simulink model "ANTIGOcontrolador"  (R2021a)
settings: Solver=ode23t  StartTime=0.0  StopTime=60  MaxStep=1e-3  RelTol=1e-3
values from neighbouring files (symbols this model uses):
  AL = double(subs(A_par))    [ANTImodeloMATEMATICOFINAL.m]
  BL = double(subs(B_par))    [ANTImodeloMATEMATICOFINAL.m]
  Blo = 8.18575752786119e-06    (= 8.18575752786e-06)    [ANTImodeloMATEMATICOFINAL.m]
  Bmo = 2.02156082362446e-07    (= 2.02156082362e-07)    [ANTImodeloMATEMATICOFINAL.m]
  CL = double(subs(C_par))    [ANTImodeloMATEMATICOFINAL.m]
  DL = double(subs(D_par))    [ANTImodeloMATEMATICOFINAL.m]
  do = 0.06862-0.021    (= 0.04762)    [ANTImodeloMATEMATICOFINAL.m]
  go = 9.81    [ANTImodeloMATEMATICOFINAL.m]
  Jlo = 0.00100697016255642    (= 0.00100697016256)    [ANTImodeloMATEMATICOFINAL.m]
  Jmo = 2.08549279330578e-07    (= 2.08549279331e-07)    [ANTImodeloMATEMATICOFINAL.m]
  Kes = K(:,1:n)    [ANTImodeloMATEMATICOFINAL.m]
  Ki = -K(:,n+1:end)    [ANTImodeloMATEMATICOFINAL.m]
  Kio = 0.00119530882984502    (= 0.00119530882985)    [ANTImodeloMATEMATICOFINAL.m]
  Kvo = 0.0035694528924319    (= 0.00356945289243)    [ANTImodeloMATEMATICOFINAL.m]
  Lo = 0.667669785204658    (= 0.667669785205)    [ANTImodeloMATEMATICOFINAL.m]
  mo = 0.17244    [ANTImodeloMATEMATICOFINAL.m]
  no = 120    [ANTImodeloMATEMATICOFINAL.m]
  Ro = 5.15610211779038    (= 5.15610211779)    [ANTImodeloMATEMATICOFINAL.m]
  Tm = 0.03    [ANTImodeloMATEMATICOFINAL.m]
  Vin0 = Ro*X10    (= 0)    [ANTImodeloMATEMATICOFINAL.m]
  X10 = 0    [ANTImodeloMATEMATICOFINAL.m]
  X20 = 0    [ANTImodeloMATEMATICOFINAL.m]
  X30 = 0    [ANTImodeloMATEMATICOFINAL.m]
libraries: cstblocks x6, slpidlib x4
(part 1 of 2)
settings Model: Creator=hubertdelgado  LastModifiedBy=hubertdelgado

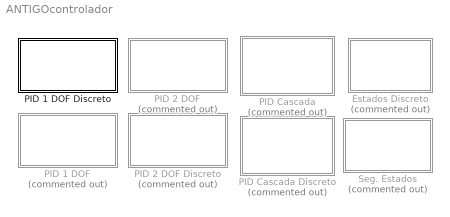
== system ANTIGOcontrolador ==
  Estados Discreto : Subsystem  Commented=on
  "PID 1 DOF " : Subsystem  Commented=on
  PID 1 DOF Discreto : Subsystem
  PID 2 DOF : Subsystem  Commented=on
  PID 2 DOF Discreto : Subsystem  Commented=on
  PID Cascada : Subsystem  Commented=on
  PID Cascada Discreto : Subsystem  Commented=on
  Seg. Estados : Subsystem  Commented=on

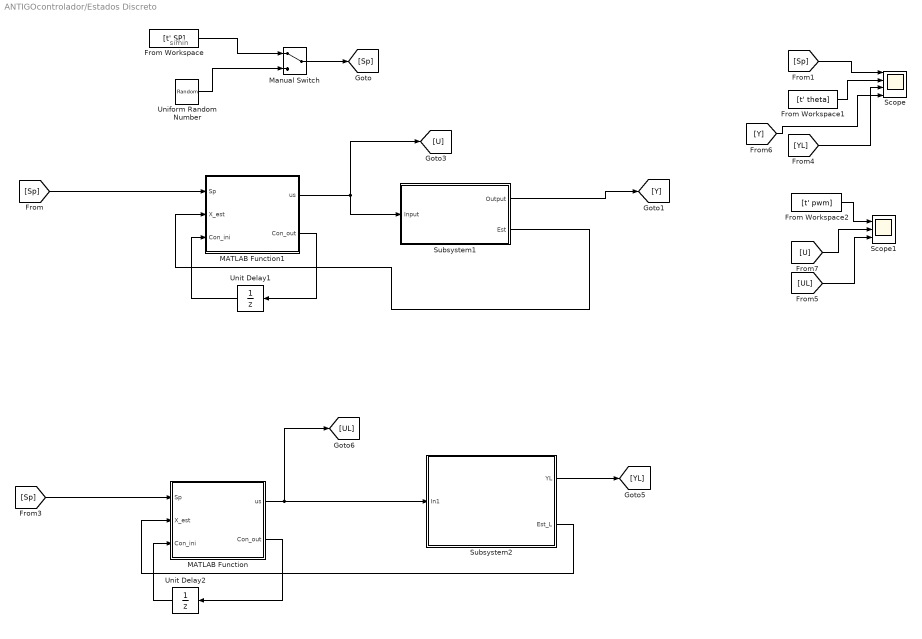
== system ANTIGOcontrolador/Estados Discreto ==
  note: simin
  From Workspace : FromWorkspace  VariableName=[t' SP]
  From Workspace1 : FromWorkspace  VariableName=[t' theta]
  From Workspace2 : FromWorkspace  VariableName=[t' pwm]
  MATLAB Function : MATLAB Function  TreatAsAtomicUnit=on
  MATLAB Function1 : MATLAB Function  TreatAsAtomicUnit=on
  Manual Switch : ManualSwitch
  Scope : Scope  NumInputPorts=4
  Scope1 : Scope  NumInputPorts=3
  Subsystem1 : Subsystem
  Subsystem2 : Subsystem
  Uniform Random Number : UniformRandomNumber  Minimum=-120*(pi/180)  Maximum=120*(pi/180)  SampleTime=10
  Unit Delay1 : UnitDelay  InitialCondition=zeros(1,2)  SampleTime=Tm  HasFrameUpgradeWarning=on
  Unit Delay2 : UnitDelay  InitialCondition=zeros(1,2)  SampleTime=Tm  HasFrameUpgradeWarning=on
  wires:
  Subsystem1/1(Output) -> [Y]
  MATLAB Function/1(us) -> Subsystem2/1(In1), [UL]
  [Sp] -> MATLAB Function/1(Sp)
  MATLAB Function/2(Con_out) -> Unit Delay2/1
  Unit Delay2/1 -> MATLAB Function/3(Con_ini)
  Subsystem2/2(Est_L) -> MATLAB Function/2(X_est)
  Subsystem2/1(YL) -> [YL]
  Manual Switch/1 -> [Sp]
  [Y] -> Scope/4
  From Workspace2/1 -> Scope1/1
  From Workspace/1 -> Manual Switch/1
  From Workspace1/1 -> Scope/2
  Uniform Random Number/1 -> Manual Switch/2
  [Sp] -> Scope/1
  [UL] -> Scope1/3
  [U] -> Scope1/2
  [YL] -> Scope/3
  Subsystem1/2(Est) -> MATLAB Function1/2(X_est)
  Unit Delay1/1 -> MATLAB Function1/3(Con_ini)
  MATLAB Function1/2(Con_out) -> Unit Delay1/1
  [Sp] -> MATLAB Function1/1(Sp)
  MATLAB Function1/1(us) -> [U], Subsystem1/1(Input)

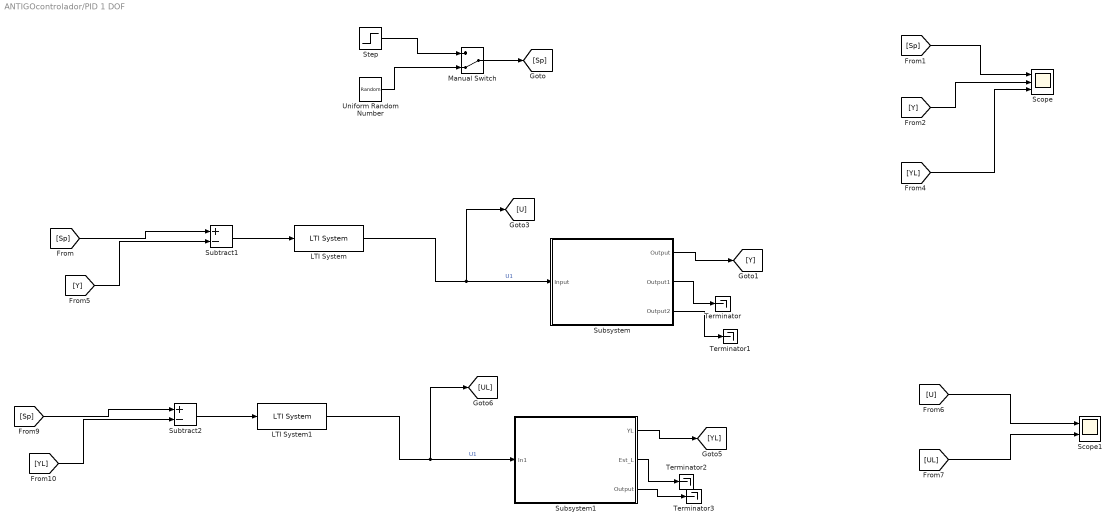
== system ANTIGOcontrolador/PID 1 DOF  ==
  LTI System : cstblocks/LTI System  sys=Cpids  IC=[]
  LTI System1 : cstblocks/LTI System  sys=Cpids  IC=[]
  Manual Switch : ManualSwitch  CurrentSetting=0
  Scope : Scope  NumInputPorts=3
  Scope1 : Scope  NumInputPorts=2
  Step : Step  Time=0  After=0  SampleTime=0
  Subsystem : Subsystem
  Subsystem1 : Subsystem
  Subtract1 : Sum  Inputs=+-
  Subtract2 : Sum  Inputs=+-
  Terminator{,1..3} (4 alike) : Terminator
  Uniform Random Number : UniformRandomNumber  Minimum=-70*(pi/180)  Maximum=70*(pi/180)  SampleTime=10
  wires:
  Manual Switch/1 -> [Sp]
  Uniform Random Number/1 -> Manual Switch/2
  [U] -> Scope1/1
  [UL] -> Scope1/2
  Step/1 -> Manual Switch/1
  Subtract1/1 -> LTI System/1
  LTI System/1 -> Subsystem/1(Input), [U]  "U1"
  [Sp] -> Subtract1/1
  [Y] -> Subtract1/2
  Subsystem/1(Output) -> [Y]
  Subtract2/1 -> LTI System1/1
  [YL] -> Subtract2/2
  LTI System1/1 -> Subsystem1/1(In1), [UL]  "U1"
  Subsystem1/2(Est_L) -> Terminator2/1
  Subsystem1/1(YL) -> [YL]
  [Sp] -> Subtract2/1
  [Sp] -> Scope/1
  [Y] -> Scope/2
  [YL] -> Scope/3
  Subsystem/2(Output1) -> Terminator/1
  Subsystem/3(Output2) -> Terminator1/1
  Subsystem1/3(Output) -> Terminator3/1

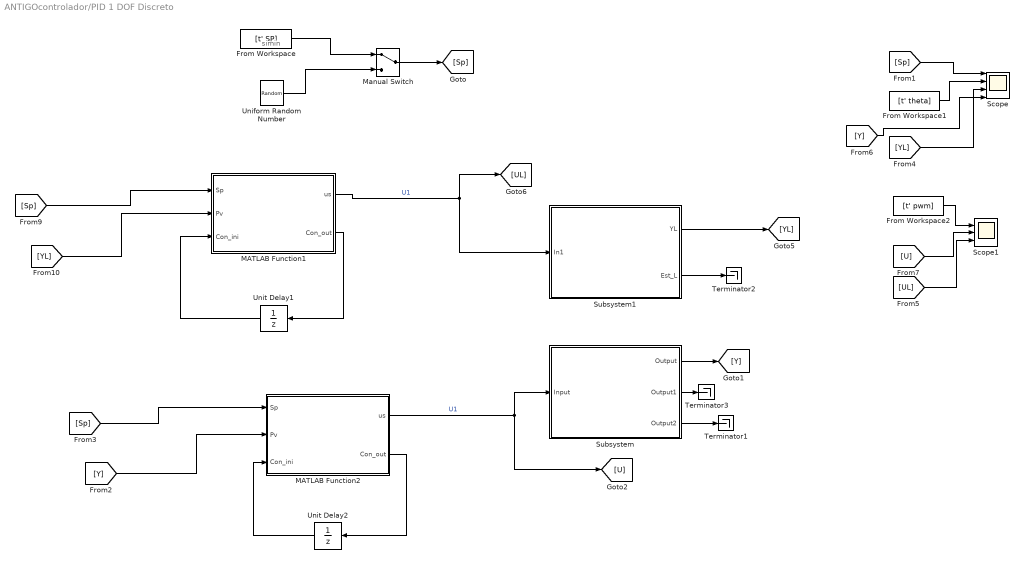
== system ANTIGOcontrolador/PID 1 DOF Discreto ==
  note: simin
  From Workspace : FromWorkspace  VariableName=[t' SP]
  From Workspace1 : FromWorkspace  VariableName=[t' theta]
  From Workspace2 : FromWorkspace  VariableName=[t' pwm]
  MATLAB Function1 : MATLAB Function  TreatAsAtomicUnit=on
  MATLAB Function2 : MATLAB Function  TreatAsAtomicUnit=on
  Manual Switch : ManualSwitch
  Scope : Scope  NumInputPorts=4
  Scope1 : Scope  NumInputPorts=3
  Subsystem : Subsystem
  Subsystem1 : Subsystem
  Terminator1 : Terminator
  Terminator2 : Terminator
  Terminator3 : Terminator
  Uniform Random Number : UniformRandomNumber  Minimum=-60*(pi/180)  Maximum=60*(pi/180)  SampleTime=10
  Unit Delay1 : UnitDelay  InitialCondition=zeros(4,1)  SampleTime=Tm  HasFrameUpgradeWarning=on
  Unit Delay2 : UnitDelay  InitialCondition=zeros(5,1)  SampleTime=Tm  HasFrameUpgradeWarning=on
  wires:
  Manual Switch/1 -> [Sp]
  Uniform Random Number/1 -> Manual Switch/2
  From Workspace2/1 -> Scope1/1
  [U] -> Scope1/2
  From Workspace/1 -> Manual Switch/1
  [YL] -> MATLAB Function1/2(Pv)
  MATLAB Function1/1(us) -> Subsystem1/1(In1), [UL]  "U1"
  Subsystem1/2(Est_L) -> Terminator2/1
  Subsystem1/1(YL) -> [YL]
  [Sp] -> Scope/1
  From Workspace1/1 -> Scope/2
  [YL] -> Scope/3
  Unit Delay1/1 -> MATLAB Function1/3(Con_ini)
  [Sp] -> MATLAB Function1/1(Sp)
  MATLAB Function1/2(Con_out) -> Unit Delay1/1
  Unit Delay2/1 -> MATLAB Function2/3(Con_ini)
  MATLAB Function2/2(Con_out) -> Unit Delay2/1
  MATLAB Function2/1(us) -> [U], Subsystem/1(Input)  "U1"
  [Sp] -> MATLAB Function2/1(Sp)
  [Y] -> MATLAB Function2/2(Pv)
  Subsystem/1(Output) -> [Y]
  Subsystem/3(Output2) -> Terminator1/1
  Subsystem/2(Output1) -> Terminator3/1
  [UL] -> Scope1/3
  [Y] -> Scope/4

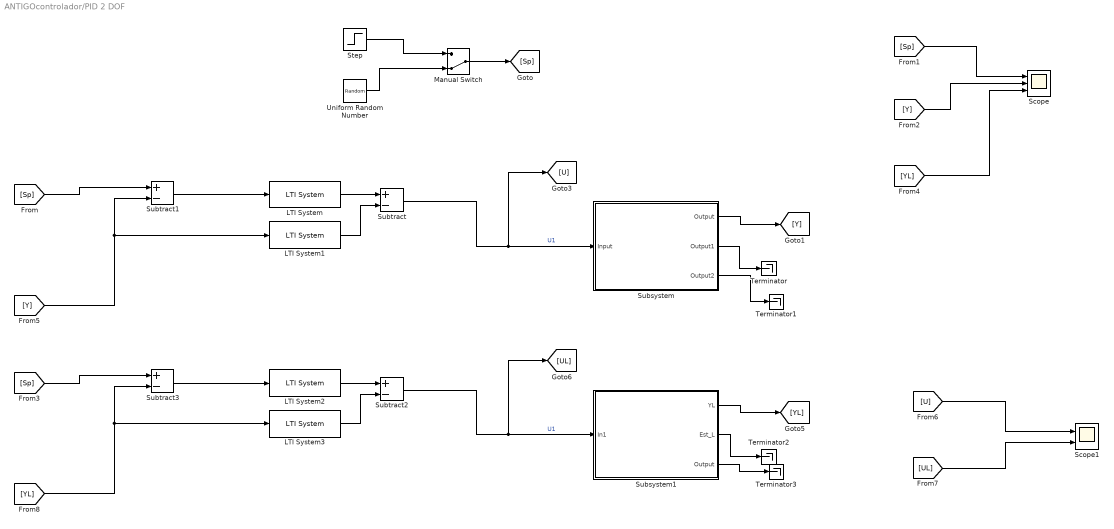
== system ANTIGOcontrolador/PID 2 DOF ==
  LTI System : cstblocks/LTI System  sys=C1s  IC=[]
  LTI System1 : cstblocks/LTI System  sys=C2s  IC=[]
  LTI System2 : cstblocks/LTI System  sys=C1s  IC=[]
  LTI System3 : cstblocks/LTI System  sys=C2s  IC=[]
  Manual Switch : ManualSwitch  CurrentSetting=0
  Scope : Scope  NumInputPorts=3
  Scope1 : Scope  NumInputPorts=2
  Step : Step  Time=0  After=0  SampleTime=0
  Subsystem : Subsystem
  Subsystem1 : Subsystem
  Subtract{,1..3} (4 alike) : Sum  Inputs=+-
  Terminator{,1..3} (4 alike) : Terminator
  Uniform Random Number : UniformRandomNumber  Minimum=-60*(pi/180)  Maximum=60*(pi/180)  SampleTime=10
  wires:
  LTI System/1 -> Subtract/1
  Subtract1/1 -> LTI System/1
  [Sp] -> Subtract1/1
  [Y] -> LTI System1/1, Subtract1/2
  LTI System1/1 -> Subtract/2
  Subtract2/1 -> Subsystem1/1(In1), [UL]  "U1"
  Subsystem1/3(Output) -> Terminator3/1
  Subtract/1 -> Subsystem/1(Input), [U]  "U1"
  Subsystem1/2(Est_L) -> Terminator2/1
  Subsystem/3(Output2) -> Terminator1/1
  Subsystem1/1(YL) -> [YL]
  Subsystem/2(Output1) -> Terminator/1
  Subsystem/1(Output) -> [Y]
  [Sp] -> Subtract3/1
  LTI System3/1 -> Subtract2/2
  LTI System2/1 -> Subtract2/1
  Subtract3/1 -> LTI System2/1
  [YL] -> LTI System3/1, Subtract3/2
  [UL] -> Scope1/2
  Step/1 -> Manual Switch/1
  Manual Switch/1 -> [Sp]
  [Y] -> Scope/2
  [Sp] -> Scope/1
  [YL] -> Scope/3
  [U] -> Scope1/1
  Uniform Random Number/1 -> Manual Switch/2

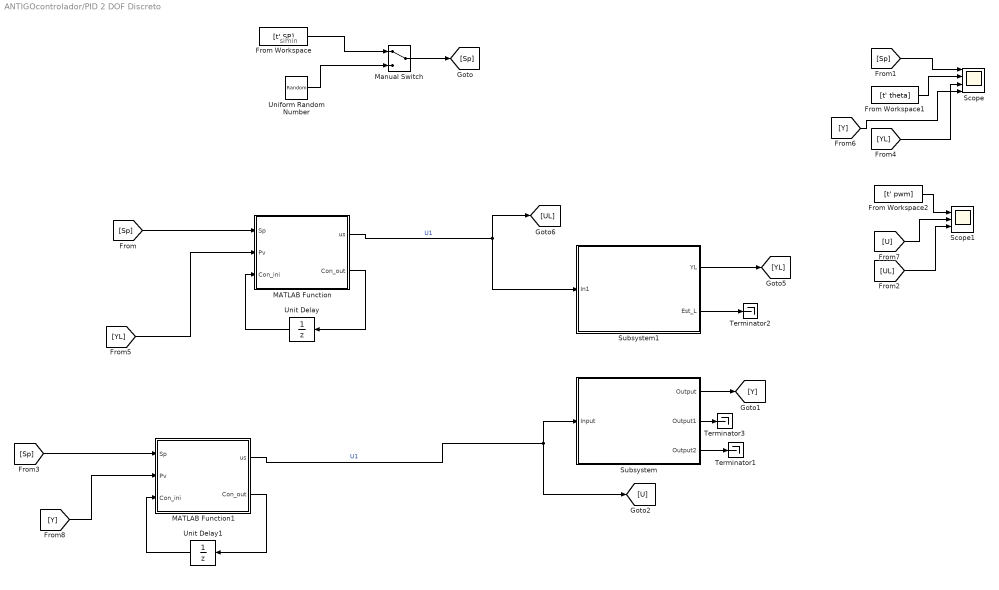
== system ANTIGOcontrolador/PID 2 DOF Discreto ==
  note: simin
  From Workspace : FromWorkspace  VariableName=[t' SP]
  From Workspace1 : FromWorkspace  VariableName=[t' theta]
  From Workspace2 : FromWorkspace  VariableName=[t' pwm]
  MATLAB Function : MATLAB Function  TreatAsAtomicUnit=on
  MATLAB Function1 : MATLAB Function  TreatAsAtomicUnit=on
  Manual Switch : ManualSwitch
  Scope : Scope  NumInputPorts=4
  Scope1 : Scope  NumInputPorts=3
  Subsystem : Subsystem
  Subsystem1 : Subsystem
  Terminator1 : Terminator
  Terminator2 : Terminator
  Terminator3 : Terminator
  Uniform Random Number : UniformRandomNumber  Minimum=-65*(pi/180)  Maximum=65*(pi/180)  SampleTime=10
  Unit Delay : UnitDelay  InitialCondition=zeros(6,1)  SampleTime=Tm  HasFrameUpgradeWarning=on
  Unit Delay1 : UnitDelay  InitialCondition=zeros(6,1)  SampleTime=Tm  HasFrameUpgradeWarning=on
  wires:
  [Sp] -> MATLAB Function/1(Sp)
  Unit Delay/1 -> MATLAB Function/3(Con_ini)
  MATLAB Function/2(Con_out) -> Unit Delay/1
  From Workspace1/1 -> Scope/2
  [YL] -> Scope/3
  [UL] -> Scope1/3
  [U] -> Scope1/2
  [Sp] -> Scope/1
  Uniform Random Number/1 -> Manual Switch/2
  From Workspace/1 -> Manual Switch/1
  From Workspace2/1 -> Scope1/1
  Manual Switch/1 -> [Sp]
  [Y] -> Scope/4
  Subsystem/2(Output1) -> Terminator3/1
  MATLAB Function/1(us) -> Subsystem1/1(In1), [UL]  "U1"
  Subsystem1/2(Est_L) -> Terminator2/1
  Subsystem1/1(YL) -> [YL]
  Subsystem/3(Output2) -> Terminator1/1
  Subsystem/1(Output) -> [Y]
  MATLAB Function1/1(us) -> [U], Subsystem/1(Input)  "U1"
  [Sp] -> MATLAB Function1/1(Sp)
  Unit Delay1/1 -> MATLAB Function1/3(Con_ini)
  MATLAB Function1/2(Con_out) -> Unit Delay1/1
  [YL] -> MATLAB Function/2(Pv)
  [Y] -> MATLAB Function1/2(Pv)

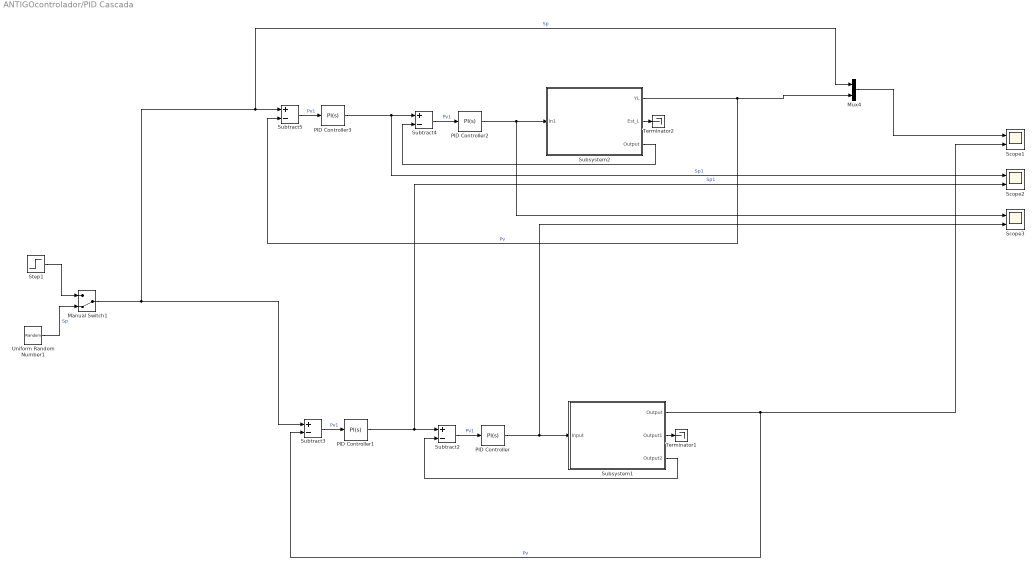
== system ANTIGOcontrolador/PID Cascada ==
  Manual Switch1 : ManualSwitch  CurrentSetting=0
  Mux4 : Mux  Inputs=2
  PID Controller : slpidlib/PID Controller  Controller=PI  Form=Parallel  TimeDomain=Continuous-time  UseExternalTs=off  SampleTime=-1  IntegratorMethod=Forward Euler  FilterMethod=Forward Euler  ControllerParametersSource=internal  P=0.439531738224972  I=0.0931065859182185  D=35.8399189335653  UseFilter=on  N=15672.9006565225  TunerSelectOption=Transfer Function Based (PID Tuner App)  InitialConditionSource=internal  InitialConditionForIntegrator=0  InitialConditionForFilter=0  DifferentiatorICPrevScaledInput=0  ExternalReset=none  TrackingMode=off  Kt=1  LimitOutput=on  SatLimitsSource=internal  UpperSaturationLimit=100  LowerSaturationLimit=-100  LinearizeAsGain=on  AntiWindupMode=none  Kb=1  POutMin=[]  POutMax=[]  IOutMin=[]  IOutMax=[]  DOutMin=[]  DOutMax=[]  NOutMin=[]  NOutMax=[]  SumOutMin=[]  SumOutMax=[]  SaturationOutMin=[]  SaturationOutMax=[]  PParamMin=[]  PParamMax=[]  IParamMin=[]  IParamMax=[]  DParamMin=[]  DParamMax=[]  NParamMin=[]  NParamMax=[]  KbParamMin=[]  KbParamMax=[]  KtParamMin=[]  KtParamMax=[]  KbOutMin=[]  KbOutMax=[]  KtOutMin=[]  KtOutMax=[]  IntegratorOutMin=[]  IntegratorOutMax=[]  FilterOutMin=[]  FilterOutMax=[]  SumI1OutMin=[]  SumI1OutMax=[]  SumI2OutMin=[]  SumI2OutMax=[]  SumI3OutMin=[]  SumI3OutMax=[]  SumI4OutMin=[]  SumI4OutMax=[]  SumDOutMin=[]  SumDOutMax=[]  DifferentiatorOutMin=[]  DifferentiatorOutMax=[]  FilterDiffOutCoefMin=[]  FilterDiffOutCoefMax=[]  ReciprocalOutMin=[]  ReciprocalOutMax=[]  SumDenOutMin=[]  SumDenOutMax=[]  SumNumOutMin=[]  SumNumOutMax=[]  DivideOutMin=[]  DivideOutMax=[]  UdiffTsProdOutMin=[]  UdiffTsProdOutMax=[]  NTsProdOutMin=[]  NTsProdOutMax=[]  UintegralTsProdOutMin=[]  UintegralTsProdOutMax=[]  UngainTsProdOutMin=[]  UngainTsProdOutMax=[]  IntegratorContinuousStateAttributes=''  IntegratorStateMustResolveToSignalObject=off  IntegratorRTWStateStorageClass=Auto  FilterContinuousStateAttributes=''  FilterStateMustResolveToSignalObject=off  FilterRTWStateStorageClass=Auto  ParallelPVariant=InternalParameters  IdealPVariant=Disabled  IVariant=InternalParameters  DVariant=Disabled  IntegratorVariant=Continuous  SatVariant=Enabled  AWVariant=Passthrough  PCopyVariant=Disabled  TRVariant=Disabled  FdbkBlocksVariant=Forward  IdealPFdbkVariant=Disabled  SatFdbkVariant=Disabled  DerivativeFilterVariant=Disabled  NVariant=Disabled  NCopyVariant=Disabled_SignalSpec  FilterICVariant=Disabled  IntegratorICVariant=InternalICs  ExternalResetVariant=Disabled  TRSumVariant=Passthrough  SumFdbkVariant=Disabled  SumVariant=Sum_PI  TsampFilterVariant=InternalTs  TsampNgainVariant=Passthrough  TsampIntegralVariant=Passthrough  ExternalSaturationOutDataTypeStr=Inherit: Same as second input
  PID Controller1 : slpidlib/PID Controller  Controller=PI  Form=Parallel  TimeDomain=Continuous-time  UseExternalTs=off  SampleTime=-1  IntegratorMethod=Forward Euler  FilterMethod=Forward Euler  ControllerParametersSource=internal  P=0  I=93.1384599522807  D=0.271518816024789  UseFilter=on  N=3961.125137588  TunerSelectOption=Transfer Function Based (PID Tuner App)  InitialConditionSource=internal  InitialConditionForIntegrator=0  InitialConditionForFilter=0  DifferentiatorICPrevScaledInput=0  ExternalReset=none  TrackingMode=off  Kt=1  LimitOutput=on  SatLimitsSource=internal  UpperSaturationLimit=40  LowerSaturationLimit=-40  LinearizeAsGain=on  AntiWindupMode=none  Kb=1  POutMin=[]  POutMax=[]  IOutMin=[]  IOutMax=[]  DOutMin=[]  DOutMax=[]  NOutMin=[]  NOutMax=[]  SumOutMin=[]  SumOutMax=[]  SaturationOutMin=[]  SaturationOutMax=[]  PParamMin=[]  PParamMax=[]  IParamMin=[]  IParamMax=[]  DParamMin=[]  DParamMax=[]  NParamMin=[]  NParamMax=[]  KbParamMin=[]  KbParamMax=[]  KtParamMin=[]  KtParamMax=[]  KbOutMin=[]  KbOutMax=[]  KtOutMin=[]  KtOutMax=[]  IntegratorOutMin=[]  IntegratorOutMax=[]  FilterOutMin=[]  FilterOutMax=[]  SumI1OutMin=[]  SumI1OutMax=[]  SumI2OutMin=[]  SumI2OutMax=[]  SumI3OutMin=[]  SumI3OutMax=[]  SumI4OutMin=[]  SumI4OutMax=[]  SumDOutMin=[]  SumDOutMax=[]  DifferentiatorOutMin=[]  DifferentiatorOutMax=[]  FilterDiffOutCoefMin=[]  FilterDiffOutCoefMax=[]  ReciprocalOutMin=[]  ReciprocalOutMax=[]  SumDenOutMin=[]  SumDenOutMax=[]  SumNumOutMin=[]  SumNumOutMax=[]  DivideOutMin=[]  DivideOutMax=[]  UdiffTsProdOutMin=[]  UdiffTsProdOutMax=[]  NTsProdOutMin=[]  NTsProdOutMax=[]  UintegralTsProdOutMin=[]  UintegralTsProdOutMax=[]  UngainTsProdOutMin=[]  UngainTsProdOutMax=[]  IntegratorContinuousStateAttributes=''  IntegratorStateMustResolveToSignalObject=off  IntegratorRTWStateStorageClass=Auto  FilterContinuousStateAttributes=''  FilterStateMustResolveToSignalObject=off  FilterRTWStateStorageClass=Auto  ParallelPVariant=InternalParameters  IdealPVariant=Disabled  IVariant=InternalParameters  DVariant=Disabled  IntegratorVariant=Continuous  SatVariant=Enabled  AWVariant=Passthrough  PCopyVariant=Disabled  TRVariant=Disabled  FdbkBlocksVariant=Forward  IdealPFdbkVariant=Disabled  SatFdbkVariant=Disabled  DerivativeFilterVariant=Disabled  NVariant=Disabled  NCopyVariant=Disabled_SignalSpec  FilterICVariant=Disabled  IntegratorICVariant=InternalICs  ExternalResetVariant=Disabled  TRSumVariant=Passthrough  SumFdbkVariant=Disabled  SumVariant=Sum_PI  TsampFilterVariant=InternalTs  TsampNgainVariant=Passthrough  TsampIntegralVariant=Passthrough  ExternalSaturationOutDataTypeStr=Inherit: Same as second input
  PID Controller2 : slpidlib/PID Controller  Controller=PI  Form=Parallel  TimeDomain=Continuous-time  UseExternalTs=off  SampleTime=-1  IntegratorMethod=Forward Euler  FilterMethod=Forward Euler  ControllerParametersSource=internal  P=0.439531738224972  I=0.0931065859182185  D=35.8399189335653  UseFilter=on  N=15672.9006565225  TunerSelectOption=Transfer Function Based (PID Tuner App)  InitialConditionSource=internal  InitialConditionForIntegrator=0  InitialConditionForFilter=0  DifferentiatorICPrevScaledInput=0  ExternalReset=none  TrackingMode=off  Kt=1  LimitOutput=on  SatLimitsSource=internal  UpperSaturationLimit=100  LowerSaturationLimit=-100  LinearizeAsGain=on  AntiWindupMode=none  Kb=1  POutMin=[]  POutMax=[]  IOutMin=[]  IOutMax=[]  DOutMin=[]  DOutMax=[]  NOutMin=[]  NOutMax=[]  SumOutMin=[]  SumOutMax=[]  SaturationOutMin=[]  SaturationOutMax=[]  PParamMin=[]  PParamMax=[]  IParamMin=[]  IParamMax=[]  DParamMin=[]  DParamMax=[]  NParamMin=[]  NParamMax=[]  KbParamMin=[]  KbParamMax=[]  KtParamMin=[]  KtParamMax=[]  KbOutMin=[]  KbOutMax=[]  KtOutMin=[]  KtOutMax=[]  IntegratorOutMin=[]  IntegratorOutMax=[]  FilterOutMin=[]  FilterOutMax=[]  SumI1OutMin=[]  SumI1OutMax=[]  SumI2OutMin=[]  SumI2OutMax=[]  SumI3OutMin=[]  SumI3OutMax=[]  SumI4OutMin=[]  SumI4OutMax=[]  SumDOutMin=[]  SumDOutMax=[]  DifferentiatorOutMin=[]  DifferentiatorOutMax=[]  FilterDiffOutCoefMin=[]  FilterDiffOutCoefMax=[]  ReciprocalOutMin=[]  ReciprocalOutMax=[]  SumDenOutMin=[]  SumDenOutMax=[]  SumNumOutMin=[]  SumNumOutMax=[]  DivideOutMin=[]  DivideOutMax=[]  UdiffTsProdOutMin=[]  UdiffTsProdOutMax=[]  NTsProdOutMin=[]  NTsProdOutMax=[]  UintegralTsProdOutMin=[]  UintegralTsProdOutMax=[]  UngainTsProdOutMin=[]  UngainTsProdOutMax=[]  IntegratorContinuousStateAttributes=''  IntegratorStateMustResolveToSignalObject=off  IntegratorRTWStateStorageClass=Auto  FilterContinuousStateAttributes=''  FilterStateMustResolveToSignalObject=off  FilterRTWStateStorageClass=Auto  ParallelPVariant=InternalParameters  IdealPVariant=Disabled  IVariant=InternalParameters  DVariant=Disabled  IntegratorVariant=Continuous  SatVariant=Enabled  AWVariant=Passthrough  PCopyVariant=Disabled  TRVariant=Disabled  FdbkBlocksVariant=Forward  IdealPFdbkVariant=Disabled  SatFdbkVariant=Disabled  DerivativeFilterVariant=Disabled  NVariant=Disabled  NCopyVariant=Disabled_SignalSpec  FilterICVariant=Disabled  IntegratorICVariant=InternalICs  ExternalResetVariant=Disabled  TRSumVariant=Passthrough  SumFdbkVariant=Disabled  SumVariant=Sum_PI  TsampFilterVariant=InternalTs  TsampNgainVariant=Passthrough  TsampIntegralVariant=Passthrough  ExternalSaturationOutDataTypeStr=Inherit: Same as second input
  PID Controller3 : slpidlib/PID Controller  Controller=PI  Form=Parallel  TimeDomain=Continuous-time  UseExternalTs=off  SampleTime=-1  IntegratorMethod=Forward Euler  FilterMethod=Forward Euler  ControllerParametersSource=internal  P=0  I=93.1384599522807  D=0.271518816024789  UseFilter=on  N=3961.125137588  TunerSelectOption=Transfer Function Based (PID Tuner App)  InitialConditionSource=internal  InitialConditionForIntegrator=0  InitialConditionForFilter=0  DifferentiatorICPrevScaledInput=0  ExternalReset=none  TrackingMode=off  Kt=1  LimitOutput=on  SatLimitsSource=internal  UpperSaturationLimit=40  LowerSaturationLimit=-40  LinearizeAsGain=on  AntiWindupMode=none  Kb=1  POutMin=[]  POutMax=[]  IOutMin=[]  IOutMax=[]  DOutMin=[]  DOutMax=[]  NOutMin=[]  NOutMax=[]  SumOutMin=[]  SumOutMax=[]  SaturationOutMin=[]  SaturationOutMax=[]  PParamMin=[]  PParamMax=[]  IParamMin=[]  IParamMax=[]  DParamMin=[]  DParamMax=[]  NParamMin=[]  NParamMax=[]  KbParamMin=[]  KbParamMax=[]  KtParamMin=[]  KtParamMax=[]  KbOutMin=[]  KbOutMax=[]  KtOutMin=[]  KtOutMax=[]  IntegratorOutMin=[]  IntegratorOutMax=[]  FilterOutMin=[]  FilterOutMax=[]  SumI1OutMin=[]  SumI1OutMax=[]  SumI2OutMin=[]  SumI2OutMax=[]  SumI3OutMin=[]  SumI3OutMax=[]  SumI4OutMin=[]  SumI4OutMax=[]  SumDOutMin=[]  SumDOutMax=[]  DifferentiatorOutMin=[]  DifferentiatorOutMax=[]  FilterDiffOutCoefMin=[]  FilterDiffOutCoefMax=[]  ReciprocalOutMin=[]  ReciprocalOutMax=[]  SumDenOutMin=[]  SumDenOutMax=[]  SumNumOutMin=[]  SumNumOutMax=[]  DivideOutMin=[]  DivideOutMax=[]  UdiffTsProdOutMin=[]  UdiffTsProdOutMax=[]  NTsProdOutMin=[]  NTsProdOutMax=[]  UintegralTsProdOutMin=[]  UintegralTsProdOutMax=[]  UngainTsProdOutMin=[]  UngainTsProdOutMax=[]  IntegratorContinuousStateAttributes=''  IntegratorStateMustResolveToSignalObject=off  IntegratorRTWStateStorageClass=Auto  FilterContinuousStateAttributes=''  FilterStateMustResolveToSignalObject=off  FilterRTWStateStorageClass=Auto  ParallelPVariant=InternalParameters  IdealPVariant=Disabled  IVariant=InternalParameters  DVariant=Disabled  IntegratorVariant=Continuous  SatVariant=Enabled  AWVariant=Passthrough  PCopyVariant=Disabled  TRVariant=Disabled  FdbkBlocksVariant=Forward  IdealPFdbkVariant=Disabled  SatFdbkVariant=Disabled  DerivativeFilterVariant=Disabled  NVariant=Disabled  NCopyVariant=Disabled_SignalSpec  FilterICVariant=Disabled  IntegratorICVariant=InternalICs  ExternalResetVariant=Disabled  TRSumVariant=Passthrough  SumFdbkVariant=Disabled  SumVariant=Sum_PI  TsampFilterVariant=InternalTs  TsampNgainVariant=Passthrough  TsampIntegralVariant=Passthrough  ExternalSaturationOutDataTypeStr=Inherit: Same as second input
  Scope1 : Scope  NumInputPorts=2
  Scope2 : Scope  NumInputPorts=2
  Scope3 : Scope  NumInputPorts=2
  Step1 : Step  Time=0  After=2*pi/180  SampleTime=0
  Subsystem1 : Subsystem
  Subsystem2 : Subsystem
  Subtract{2..5} (4 alike) : Sum  Inputs=+-
  Terminator1 : Terminator
  Terminator2 : Terminator
  Uniform Random Number1 : UniformRandomNumber  Minimum=-30*(pi/180)  Maximum=30*(pi/180)  SampleTime=15
  wires:
  Step1/1 -> Manual Switch1/1
  Subsystem1/1(Output) -> Subtract3/2, Scope1/2  "Pv"
  Uniform Random Number1/1 -> Manual Switch1/2  "Sp"
  Subsystem1/2(Output1) -> Terminator1/1
  PID Controller/1 -> Scope3/2, Subsystem1/1(Input)
  Subtract2/1 -> PID Controller/1  "Pv1"
  PID Controller1/1 -> Scope2/2, Subtract2/1  "Sp1"
  Subsystem1/3(Output2) -> Subtract2/2
  Subtract3/1 -> PID Controller1/1  "Pv1"
  Subtract5/1 -> PID Controller3/1  "Pv1"
  Mux4/1 -> Scope1/1
  Subtract4/1 -> PID Controller2/1  "Pv1"
  Subsystem2/2(Est_L) -> Terminator2/1
  Subsystem2/3(Output) -> Subtract4/2
  PID Controller2/1 -> Scope3/1, Subsystem2/1(In1)
  PID Controller3/1 -> Scope2/1, Subtract4/1  "Sp1"
  Subsystem2/1(YL) -> Subtract5/2, Mux4/2  "Pv"
  Manual Switch1/1 -> Mux4/1, Subtract5/1, Subtract3/1  "Sp"

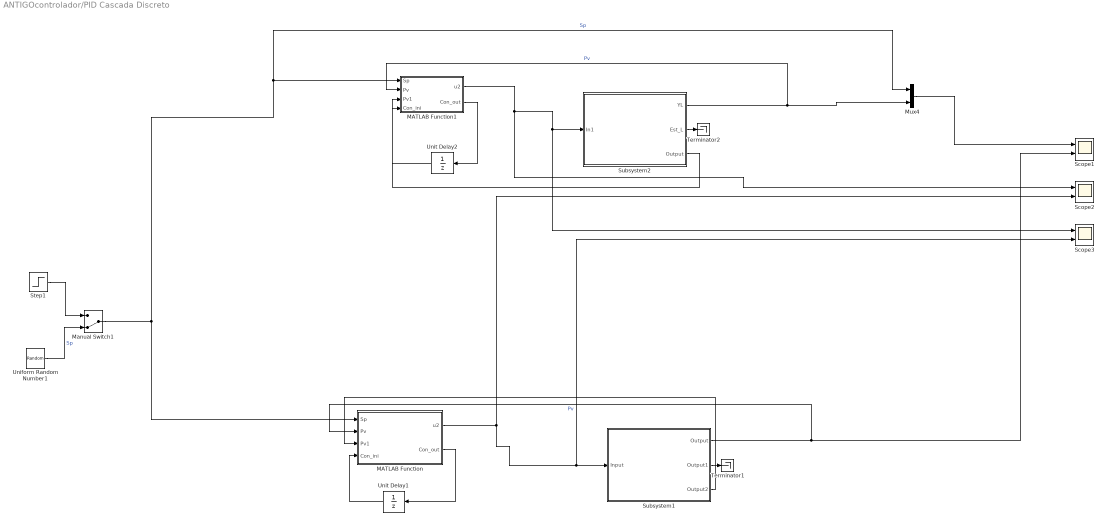
== system ANTIGOcontrolador/PID Cascada Discreto ==
  MATLAB Function : MATLAB Function  TreatAsAtomicUnit=on
  MATLAB Function1 : MATLAB Function  TreatAsAtomicUnit=on
  Manual Switch1 : ManualSwitch  CurrentSetting=0
  Mux4 : Mux  Inputs=2
  Scope1 : Scope  NumInputPorts=2
  Scope2 : Scope  NumInputPorts=2
  Scope3 : Scope  NumInputPorts=2
  Step1 : Step  Time=0  After=0*pi/180  SampleTime=0
  Subsystem1 : Subsystem
  Subsystem2 : Subsystem
  Terminator1 : Terminator
  Terminator2 : Terminator
  Uniform Random Number1 : UniformRandomNumber  Minimum=-10*(pi/180)  Maximum=10*(pi/180)  SampleTime=15
  Unit Delay1 : UnitDelay  InitialCondition=zeros(4,1)  SampleTime=Tm  HasFrameUpgradeWarning=on
  Unit Delay2 : UnitDelay  InitialCondition=zeros(4,1)  SampleTime=Tm  HasFrameUpgradeWarning=on
  wires:
  Step1/1 -> Manual Switch1/1
  Subsystem1/1(Output) -> MATLAB Function/2(Pv), Scope1/2  "Pv"
  Uniform Random Number1/1 -> Manual Switch1/2  "Sp"
  Subsystem1/2(Output1) -> Terminator1/1
  MATLAB Function/1(u2) -> Scope3/2, Subsystem1/1(Input), Scope2/2
  Mux4/1 -> Scope1/1
  Subsystem2/2(Est_L) -> Terminator2/1
  MATLAB Function1/1(u2) -> Scope2/1, Scope3/1, Subsystem2/1(In1)
  Subsystem2/1(YL) -> MATLAB Function1/2(Pv), Mux4/2  "Pv"
  Subsystem2/3(Output) -> MATLAB Function1/3(Pv1)
  MATLAB Function1/2(Con_out) -> Unit Delay2/1
  MATLAB Function/2(Con_out) -> Unit Delay1/1
  Manual Switch1/1 -> MATLAB Function/1(Sp), Mux4/1, MATLAB Function1/1(Sp)  "Sp"
  Subsystem1/3(Output2) -> MATLAB Function/3(Pv1)
  Unit Delay1/1 -> MATLAB Function/4(Con_ini)
  Unit Delay2/1 -> MATLAB Function1/4(Con_ini)

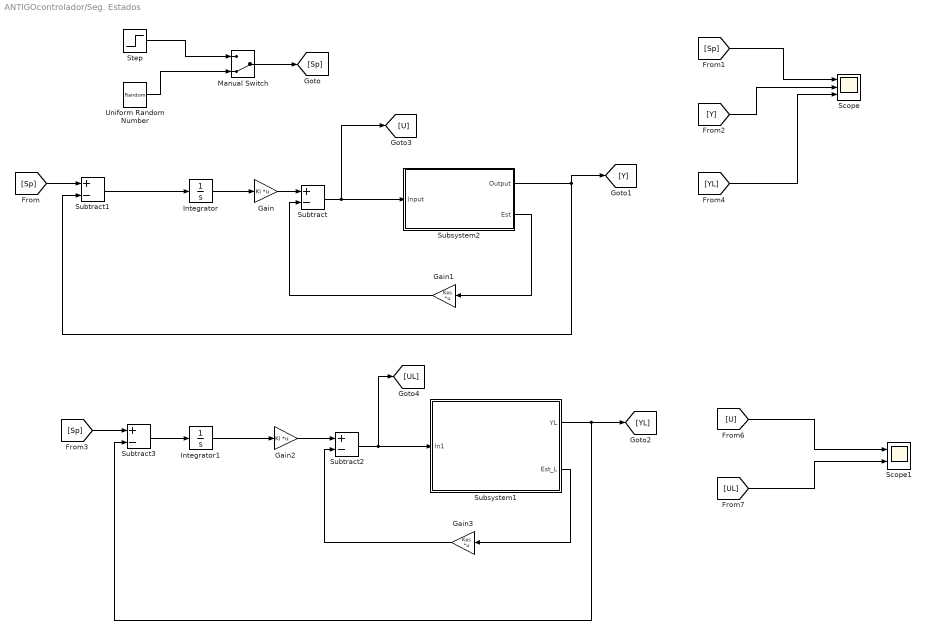
== system ANTIGOcontrolador/Seg. Estados ==
  Gain : Gain  Gain=Ki  Multiplication=Matrix(K*u)
  Gain1 : Gain  Gain=Kes  Multiplication=Matrix(K*u)
  Gain2 : Gain  Gain=Ki  Multiplication=Matrix(K*u)
  Gain3 : Gain  Gain=Kes  Multiplication=Matrix(K*u)
  Integrator : Integrator
  Integrator1 : Integrator
  Manual Switch : ManualSwitch  CurrentSetting=0
  Scope : Scope  NumInputPorts=3
  Scope1 : Scope  NumInputPorts=2
  Step : Step  Time=0  After=0  SampleTime=0
  Subsystem1 : Subsystem
  Subsystem2 : Subsystem
  Subtract{,1..3} (4 alike) : Sum  Inputs=+-
  Uniform Random Number : UniformRandomNumber  Minimum=-120*(pi/180)  Maximum=120*(pi/180)  SampleTime=10
  wires:
  Subsystem2/1(Output) -> Subtract1/2, [Y]
  Subsystem2/2(Est) -> Gain1/1
  Subtract/1 -> Subsystem2/1(Input), [U]
  Gain1/1 -> Subtract/2
  Subtract2/1 -> [UL], Subsystem1/1(In1)
  Gain/1 -> Subtract/1
  [Sp] -> Subtract1/1
  [Sp] -> Subtract3/1
  Gain2/1 -> Subtract2/1
  Subsystem1/1(YL) -> [YL], Subtract3/2
  Subsystem1/2(Est_L) -> Gain3/1
  Gain3/1 -> Subtract2/2
  Integrator/1 -> Gain/1
  Subtract1/1 -> Integrator/1
  Integrator1/1 -> Gain2/1
  Subtract3/1 -> Integrator1/1
  [UL] -> Scope1/2
  Step/1 -> Manual Switch/1
  Manual Switch/1 -> [Sp]
  [Y] -> Scope/2
  [Sp] -> Scope/1
  [YL] -> Scope/3
  [U] -> Scope1/1
  Uniform Random Number/1 -> Manual Switch/2

== system ANTIGOcontrolador/Estados Discreto/Subsystem1 ==
  Input : Inport
  Add : Sum
  Constant : Constant  Value=[Ro,Lo,Kio, Kvo, Jmo, Jlo, Bmo, Blo, no, go, do, mo]
  Constant1 : Constant  Value=Vin0
  Constant2 : Constant  Value=[X10; X20]
  Gain1 : Gain  Gain=CL  Multiplication=Matrix(K*u)
  Integrator : Integrator  InitialCondition=[X10; X20]
  MATLAB Function : MATLAB Function  TreatAsAtomicUnit=on
  Subtract1 : Sum  Inputs=+-
  Output : Outport
  Est : Outport  Port=2
  wires:
  Add/1 -> MATLAB Function/2(PWM)
  Constant2/1 -> Subtract1/2
  Constant1/1 -> Add/1
  Input/1 -> Add/2
  MATLAB Function/1(dx) -> Integrator/1
  Constant/1 -> MATLAB Function/3(parametros)
  Integrator/1 -> Subtract1/1, MATLAB Function/1(x)
  Subtract1/1 -> Est/1, Gain1/1
  Gain1/1 -> Output/1

== system ANTIGOcontrolador/Estados Discreto/Subsystem2 ==
  In1 : Inport
  Add : Sum
  Add1 : Sum
  Gain : Gain  Gain=CL  Multiplication=Matrix(K*u)
  Gain1 : Gain  Gain=AL  Multiplication=Matrix(K*u)
  Gain2 : Gain  Gain=DL  Multiplication=Matrix(K*u)
  Gain3 : Gain  Gain=BL  Multiplication=Matrix(K*u)
  Integrator : Integrator
  YL : Outport
  Est_L : Outport  Port=2
  wires:
  Gain/1 -> Add/2
  Integrator/1 -> Gain/1, Est_L/1, Gain1/1
  Add1/1 -> Integrator/1
  Gain1/1 -> Add1/2
  Gain2/1 -> Add/1
  Gain3/1 -> Add1/1
  Add/1 -> YL/1
  In1/1 -> Gain2/1, Gain3/1

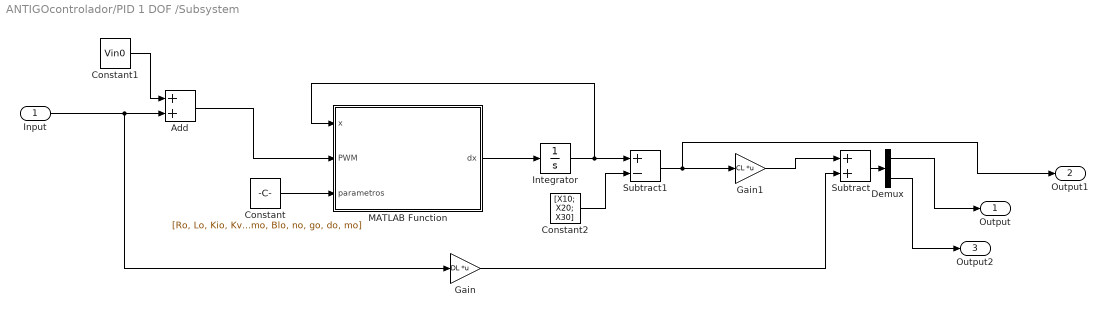
== system ANTIGOcontrolador/PID 1 DOF /Subsystem ==
  Input : Inport
  Add : Sum
  Constant : Constant  Value=[Ro, Lo, Kio, Kvo, Jmo, Jlo, Bmo, Blo, no, go, do, mo]
  Constant1 : Constant  Value=Vin0
  Constant2 : Constant  Value=[X10; X20; X30]
  Demux : Demux  Outputs=2
  Gain : Gain  Gain=DL  Multiplication=Matrix(K*u)
  Gain1 : Gain  Gain=CL  Multiplication=Matrix(K*u)
  Integrator : Integrator  InitialCondition=[X10; X20; X30]
  MATLAB Function : MATLAB Function  TreatAsAtomicUnit=on
  Subtract : Sum
  Subtract1 : Sum  Inputs=+-
  Output : Outport
  Output1 : Outport  Port=2
  Output2 : Outport  Port=3
  wires:
  Integrator/1 -> Subtract1/1, MATLAB Function/1(x)
  Add/1 -> MATLAB Function/2(PWM)
  Subtract1/1 -> Output1/1, Gain1/1
  MATLAB Function/1(dx) -> Integrator/1
  Constant1/1 -> Add/1
  Constant2/1 -> Subtract1/2
  Constant/1 -> MATLAB Function/3(parametros)
  Gain1/1 -> Subtract/1
  Gain/1 -> Subtract/2
  Input/1 -> Gain/1, Add/2
  Subtract/1 -> Demux/1
  Demux/1 -> Output/1
  Demux/2 -> Output2/1

== system ANTIGOcontrolador/PID 1 DOF /Subsystem1 ==
  In1 : Inport
  Add : Sum
  Add1 : Sum
  Demux : Demux  Outputs=2
  Gain : Gain  Gain=CL  Multiplication=Matrix(K*u)
  Gain1 : Gain  Gain=AL  Multiplication=Matrix(K*u)
  Gain2 : Gain  Gain=DL  Multiplication=Matrix(K*u)
  Gain3 : Gain  Gain=BL  Multiplication=Matrix(K*u)
  Integrator : Integrator
  YL : Outport
  Est_L : Outport  Port=2
  Output : Outport  Port=3
  wires:
  Gain/1 -> Add/2
  Integrator/1 -> Gain/1, Est_L/1, Gain1/1
  Add1/1 -> Integrator/1
  Gain1/1 -> Add1/2
  Gain2/1 -> Add/1
  Gain3/1 -> Add1/1
  In1/1 -> Gain2/1, Gain3/1
  Add/1 -> Demux/1
  Demux/1 -> YL/1
  Demux/2 -> Output/1

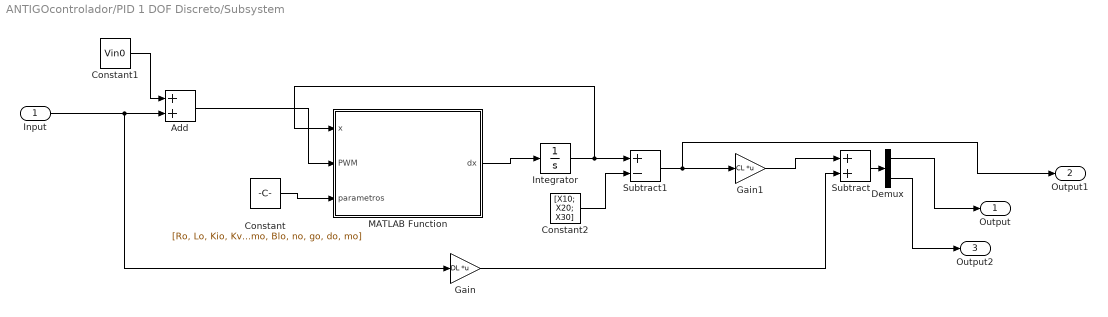
== system ANTIGOcontrolador/PID 1 DOF Discreto/Subsystem ==
  Input : Inport
  Add : Sum
  Constant : Constant  Value=[Ro, Lo, Kio, Kvo, Jmo, Jlo, Bmo, Blo, no, go, do, mo]
  Constant1 : Constant  Value=Vin0
  Constant2 : Constant  Value=[X10; X20; X30]
  Demux : Demux  Outputs=2
  Gain : Gain  Gain=DL  Multiplication=Matrix(K*u)
  Gain1 : Gain  Gain=CL  Multiplication=Matrix(K*u)
  Integrator : Integrator  InitialCondition=[X10; X20; X30]
  MATLAB Function : MATLAB Function  TreatAsAtomicUnit=on
  Subtract : Sum
  Subtract1 : Sum  Inputs=+-
  Output : Outport
  Output1 : Outport  Port=2
  Output2 : Outport  Port=3
  wires:
  Integrator/1 -> Subtract1/1, MATLAB Function/1(x)
  Add/1 -> MATLAB Function/2(PWM)
  Subtract1/1 -> Output1/1, Gain1/1
  MATLAB Function/1(dx) -> Integrator/1
  Constant1/1 -> Add/1
  Constant2/1 -> Subtract1/2
  Constant/1 -> MATLAB Function/3(parametros)
  Gain1/1 -> Subtract/1
  Gain/1 -> Subtract/2
  Input/1 -> Gain/1, Add/2
  Subtract/1 -> Demux/1
  Demux/1 -> Output/1
  Demux/2 -> Output2/1

== system ANTIGOcontrolador/PID 1 DOF Discreto/Subsystem1 ==
  In1 : Inport
  Add : Sum
  Add1 : Sum
  Demux : Demux  Outputs=2
  Gain : Gain  Gain=CL  Multiplication=Matrix(K*u)
  Gain1 : Gain  Gain=AL  Multiplication=Matrix(K*u)
  Gain2 : Gain  Gain=DL  Multiplication=Matrix(K*u)
  Gain3 : Gain  Gain=BL  Multiplication=Matrix(K*u)
  Integrator : Integrator
  Terminator : Terminator
  YL : Outport
  Est_L : Outport  Port=2
  wires:
  Gain/1 -> Add/2
  Integrator/1 -> Gain/1, Est_L/1, Gain1/1
  Add1/1 -> Integrator/1
  Gain1/1 -> Add1/2
  Gain2/1 -> Add/1
  Gain3/1 -> Add1/1
  In1/1 -> Gain2/1, Gain3/1
  Add/1 -> Demux/1
  Demux/1 -> YL/1
  Demux/2 -> Terminator/1

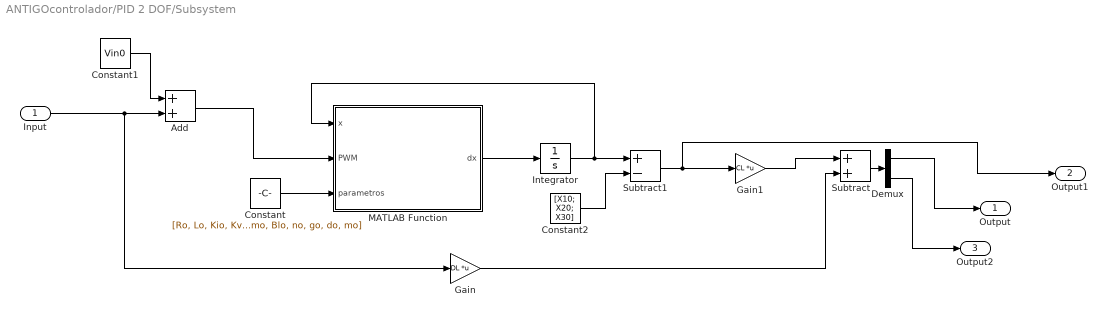
== system ANTIGOcontrolador/PID 2 DOF/Subsystem ==
  Input : Inport
  Add : Sum
  Constant : Constant  Value=[Ro, Lo, Kio, Kvo, Jmo, Jlo, Bmo, Blo, no, go, do, mo]
  Constant1 : Constant  Value=Vin0
  Constant2 : Constant  Value=[X10; X20; X30]
  Demux : Demux  Outputs=2
  Gain : Gain  Gain=DL  Multiplication=Matrix(K*u)
  Gain1 : Gain  Gain=CL  Multiplication=Matrix(K*u)
  Integrator : Integrator  InitialCondition=[X10; X20; X30]
  MATLAB Function : MATLAB Function  TreatAsAtomicUnit=on
  Subtract : Sum
  Subtract1 : Sum  Inputs=+-
  Output : Outport
  Output1 : Outport  Port=2
  Output2 : Outport  Port=3
  wires:
  Integrator/1 -> Subtract1/1, MATLAB Function/1(x)
  Add/1 -> MATLAB Function/2(PWM)
  Subtract1/1 -> Output1/1, Gain1/1
  MATLAB Function/1(dx) -> Integrator/1
  Constant1/1 -> Add/1
  Constant2/1 -> Subtract1/2
  Constant/1 -> MATLAB Function/3(parametros)
  Gain1/1 -> Subtract/1
  Gain/1 -> Subtract/2
  Input/1 -> Gain/1, Add/2
  Subtract/1 -> Demux/1
  Demux/1 -> Output/1
  Demux/2 -> Output2/1

== system ANTIGOcontrolador/PID 2 DOF/Subsystem1 ==
  In1 : Inport
  Add : Sum
  Add1 : Sum
  Demux : Demux  Outputs=2
  Gain : Gain  Gain=CL  Multiplication=Matrix(K*u)
  Gain1 : Gain  Gain=AL  Multiplication=Matrix(K*u)
  Gain2 : Gain  Gain=DL  Multiplication=Matrix(K*u)
  Gain3 : Gain  Gain=BL  Multiplication=Matrix(K*u)
  Integrator : Integrator
  YL : Outport
  Est_L : Outport  Port=2
  Output : Outport  Port=3
  wires:
  Gain/1 -> Add/2
  Integrator/1 -> Gain/1, Est_L/1, Gain1/1
  Add1/1 -> Integrator/1
  Gain1/1 -> Add1/2
  Gain2/1 -> Add/1
  Gain3/1 -> Add1/1
  In1/1 -> Gain2/1, Gain3/1
  Add/1 -> Demux/1
  Demux/1 -> YL/1
  Demux/2 -> Output/1

== system ANTIGOcontrolador/PID 2 DOF Discreto/Subsystem ==
  Input : Inport
  Add : Sum
  Constant : Constant  Value=[Ro, Lo, Kio, Kvo, Jmo, Jlo, Bmo, Blo, no, go, do, mo]
  Constant1 : Constant  Value=Vin0
  Constant2 : Constant  Value=[X10; X20; X30]
  Demux : Demux  Outputs=2
  Gain : Gain  Gain=DL  Multiplication=Matrix(K*u)
  Gain1 : Gain  Gain=CL  Multiplication=Matrix(K*u)
  Integrator : Integrator  InitialCondition=[X10; X20; X30]
  MATLAB Function : MATLAB Function  TreatAsAtomicUnit=on
  Subtract : Sum
  Subtract1 : Sum  Inputs=+-
  Output : Outport
  Output1 : Outport  Port=2
  Output2 : Outport  Port=3
  wires:
  Integrator/1 -> Subtract1/1, MATLAB Function/1(x)
  Add/1 -> MATLAB Function/2(PWM)
  Subtract1/1 -> Output1/1, Gain1/1
  MATLAB Function/1(dx) -> Integrator/1
  Constant1/1 -> Add/1
  Constant2/1 -> Subtract1/2
  Constant/1 -> MATLAB Function/3(parametros)
  Gain1/1 -> Subtract/1
  Gain/1 -> Subtract/2
  Input/1 -> Gain/1, Add/2
  Subtract/1 -> Demux/1
  Demux/1 -> Output/1
  Demux/2 -> Output2/1

== system ANTIGOcontrolador/PID 2 DOF Discreto/Subsystem1 ==
  In1 : Inport
  Add : Sum
  Add1 : Sum
  Demux : Demux  Outputs=2
  Gain : Gain  Gain=CL  Multiplication=Matrix(K*u)
  Gain1 : Gain  Gain=AL  Multiplication=Matrix(K*u)
  Gain2 : Gain  Gain=DL  Multiplication=Matrix(K*u)
  Gain3 : Gain  Gain=BL  Multiplication=Matrix(K*u)
  Integrator : Integrator
  Terminator : Terminator
  YL : Outport
  Est_L : Outport  Port=2
  wires:
  Gain/1 -> Add/2
  Integrator/1 -> Gain/1, Est_L/1, Gain1/1
  Add1/1 -> Integrator/1
  Gain1/1 -> Add1/2
  Gain2/1 -> Add/1
  Gain3/1 -> Add1/1
  In1/1 -> Gain2/1, Gain3/1
  Add/1 -> Demux/1
  Demux/1 -> YL/1
  Demux/2 -> Terminator/1

== system ANTIGOcontrolador/PID Cascada/Subsystem1 ==
  Input : Inport
  Add : Sum
  Constant : Constant  Value=[Ro, Lo, Kio, Kvo, Jmo, Jlo, Bmo, Blo, no, go, do, mo]
  Constant1 : Constant  Value=Vin0
  Constant2 : Constant  Value=[X10; X20; X30]
  Demux : Demux  Outputs=2
  Gain : Gain  Gain=DL  Multiplication=Matrix(K*u)
  Gain1 : Gain  Gain=CL  Multiplication=Matrix(K*u)
  Integrator : Integrator  InitialCondition=[X10; X20; X30]
  MATLAB Function : MATLAB Function  TreatAsAtomicUnit=on
  Subtract : Sum
  Subtract1 : Sum  Inputs=+-
  Output : Outport
  Output1 : Outport  Port=2
  Output2 : Outport  Port=3
  wires:
  Integrator/1 -> Subtract1/1, MATLAB Function/1(x)
  Add/1 -> MATLAB Function/2(PWM)
  Subtract1/1 -> Output1/1, Gain1/1
  MATLAB Function/1(dx) -> Integrator/1
  Constant1/1 -> Add/1
  Constant2/1 -> Subtract1/2
  Constant/1 -> MATLAB Function/3(parametros)
  Gain1/1 -> Subtract/1
  Gain/1 -> Subtract/2
  Input/1 -> Gain/1, Add/2
  Subtract/1 -> Demux/1
  Demux/1 -> Output/1
  Demux/2 -> Output2/1

== system ANTIGOcontrolador/PID Cascada/Subsystem2 ==
  In1 : Inport
  Add : Sum
  Add1 : Sum
  Demux : Demux  Outputs=2
  Gain : Gain  Gain=CL  Multiplication=Matrix(K*u)
  Gain1 : Gain  Gain=AL  Multiplication=Matrix(K*u)
  Gain2 : Gain  Gain=DL  Multiplication=Matrix(K*u)
  Gain3 : Gain  Gain=BL  Multiplication=Matrix(K*u)
  Integrator : Integrator
  YL : Outport
  Est_L : Outport  Port=2
  Output : Outport  Port=3
  wires:
  Gain/1 -> Add/2
  Integrator/1 -> Gain/1, Est_L/1, Gain1/1
  Add1/1 -> Integrator/1
  Gain1/1 -> Add1/2
  Gain2/1 -> Add/1
  Gain3/1 -> Add1/1
  In1/1 -> Gain2/1, Gain3/1
  Add/1 -> Demux/1
  Demux/1 -> YL/1
  Demux/2 -> Output/1

== system ANTIGOcontrolador/PID Cascada Discreto/Subsystem1 ==
  Input : Inport
  Add : Sum
  Constant : Constant  Value=[Ro, Lo, Kio, Kvo, Jmo, Jlo, Bmo, Blo, no, go, do, mo]
  Constant1 : Constant  Value=Vin0
  Constant2 : Constant  Value=[X10; X20; X30]
  Demux : Demux  Outputs=2
  Gain : Gain  Gain=DL  Multiplication=Matrix(K*u)
  Gain1 : Gain  Gain=CL  Multiplication=Matrix(K*u)
  Integrator : Integrator  InitialCondition=[X10; X20; X30]
  MATLAB Function : MATLAB Function  TreatAsAtomicUnit=on
  Subtract : Sum
  Subtract1 : Sum  Inputs=+-
  Output : Outport
  Output1 : Outport  Port=2
  Output2 : Outport  Port=3
  wires:
  Integrator/1 -> Subtract1/1, MATLAB Function/1(x)
  Add/1 -> MATLAB Function/2(PWM)
  Subtract1/1 -> Output1/1, Gain1/1
  MATLAB Function/1(dx) -> Integrator/1
  Constant1/1 -> Add/1
  Constant2/1 -> Subtract1/2
  Constant/1 -> MATLAB Function/3(parametros)
  Gain1/1 -> Subtract/1
  Gain/1 -> Subtract/2
  Input/1 -> Gain/1, Add/2
  Subtract/1 -> Demux/1
  Demux/1 -> Output/1
  Demux/2 -> Output2/1

== system ANTIGOcontrolador/PID Cascada Discreto/Subsystem2 ==
  In1 : Inport
  Add : Sum
  Add1 : Sum
  Demux : Demux  Outputs=2
  Gain : Gain  Gain=CL  Multiplication=Matrix(K*u)
  Gain1 : Gain  Gain=AL  Multiplication=Matrix(K*u)
  Gain2 : Gain  Gain=DL  Multiplication=Matrix(K*u)
  Gain3 : Gain  Gain=BL  Multiplication=Matrix(K*u)
  Integrator : Integrator
  YL : Outport
  Est_L : Outport  Port=2
  Output : Outport  Port=3
  wires:
  Gain/1 -> Add/2
  Integrator/1 -> Gain/1, Est_L/1, Gain1/1
  Add1/1 -> Integrator/1
  Gain1/1 -> Add1/2
  Gain2/1 -> Add/1
  Gain3/1 -> Add1/1
  In1/1 -> Gain2/1, Gain3/1
  Add/1 -> Demux/1
  Demux/1 -> YL/1
  Demux/2 -> Output/1

== system ANTIGOcontrolador/Seg. Estados/Subsystem1 ==
  In1 : Inport
  Add : Sum
  Add1 : Sum
  Gain : Gain  Gain=CL  Multiplication=Matrix(K*u)
  Gain1 : Gain  Gain=AL  Multiplication=Matrix(K*u)
  Gain2 : Gain  Gain=DL  Multiplication=Matrix(K*u)
  Gain3 : Gain  Gain=BL  Multiplication=Matrix(K*u)
  Integrator : Integrator
  YL : Outport
  Est_L : Outport  Port=2
  wires:
  Gain/1 -> Add/2
  Integrator/1 -> Gain/1, Est_L/1, Gain1/1
  Add1/1 -> Integrator/1
  Gain1/1 -> Add1/2
  Gain2/1 -> Add/1
  Gain3/1 -> Add1/1
  Add/1 -> YL/1
  In1/1 -> Gain2/1, Gain3/1

== system ANTIGOcontrolador/Seg. Estados/Subsystem2 ==
  Input : Inport
  Add : Sum
  Constant : Constant  Value=[Ro,Lo,Kio, Kvo, Jmo, Jlo, Bmo, Blo, no, go, do, mo]
  Constant1 : Constant  Value=Vin0
  Constant2 : Constant  Value=[X10; X20]
  Gain1 : Gain  Gain=CL  Multiplication=Matrix(K*u)
  Integrator : Integrator  InitialCondition=[X10; X20]
  MATLAB Function : MATLAB Function  TreatAsAtomicUnit=on
  Subtract1 : Sum  Inputs=+-
  Output : Outport
  Est : Outport  Port=2
  wires:
  Add/1 -> MATLAB Function/2(PWM)
  Constant2/1 -> Subtract1/2
  Constant1/1 -> Add/1
  Input/1 -> Add/2
  MATLAB Function/1(dx) -> Integrator/1
  Constant/1 -> MATLAB Function/3(parametros)
  Integrator/1 -> Subtract1/1, MATLAB Function/1(x)
  Subtract1/1 -> Est/1, Gain1/1
  Gain1/1 -> Output/1

== matlab function ANTIGOcontrolador/PID 1 DOF Discreto/MATLAB Function1 ==
  data: Sp input; us output; Pv input; Con_ini input; Con_out output
% function [us, Con_out] = fcn(Sp, Pv, Con_ini)
%  
% en_1 = Con_ini(1);
% en_2 = Con_ini(2);
% un_1 = Con_ini(3);
% un_2 = Con_ini(4);
% difact = Con_ini(5);
% umin = -100;
% umax = 100;
% kaw = 0.1; 
%  
% en = Sp - Pv;
% un = 52.346730287862997*en - 99.613623826288730*en_1 + 48.365148241217845*en_2 + 1.742509213223832*un_1 - 0.742509213223832*un_2 + kaw*difact;
%  
% us = un;
%  
% if un < umin 
%     us = umin;
% end
% if un > umax 
%     us = umax;
% end
%  
% en_2 = en_1;
% en_1 = en;
% un_2 = un_1;
% un_1 = un;
% difact = us - un;
%          
% Con_out = [en_1; en_2; un_1; un_2; difact];

function [us, Con_out] = fcn(Sp, Pv, Con_ini)

en_1 = Con_ini(1);
I_error_1 = Con_ini(2);
difact = Con_ini(3);
Ad_1 = Con_ini(4);

umin = -100;
umax = 100;

Kp = 12.194801852041582;
Ki = 1.836264365827931;
Kd = 58.215749090323079;
N = 0.135321750384943;
kaw=0.1; 


en = Sp - Pv;
Ap = Kp*en;
Ad = Kd*(en-en_1) + N*Ad_1;
I_error = en + I_error_1 + kaw*difact;
Ai = Ki*I_error;
un = Ap + Ai + Ad;
us = un;

if un < umin 
    us = umin;
end
if un > umax 
    us = umax;
end

en_1 = en;
I_error_1 = I_error;
difact = us - un;
Ad_1 = Ad;
      
Con_out = [en_1; I_error_1; difact; Ad_1];

== matlab function ANTIGOcontrolador/PID Cascada Discreto/Subsystem1/MATLAB Function ==
  data: x input; PWM input; dx output; parametros input
function dx = fcn(x,PWM,parametros)

%ESTADOS
x1 = x(1);
x2 = x(2);
x3 = x(3);

%Parametros
R = parametros(1);
L = parametros(2);
Ki = parametros(3);
Kv = parametros(4);
Jm = parametros(5);
Jl = parametros(6);
Bm = parametros(7);
Bl = parametros(8);
n = parametros(9);
g = parametros(10);
d = parametros(11);
m = parametros(12);

%EXPRESIONES
% Jt = Jm*n^2 +Jl;
% f1 = (1/L)*(((7*PWM)/100) - R*x1 - Kv*x2*n);
% f2 = (1/Jt)*(Ki*x1*n - (Bm*n^2 + Bl)*x2 - m*g*d*sin(x3));
% f3 = x2;

% MODELO 2 ESTADOS I TL WL  SALIDA TL WL
f1 = (((7*PWM)/100)-Kv*x3*n-R*x1)/(L); %di/dt
f2 = x3; %d0l/dt = Wl
f3 = ((Ki*x1*n)-x3*(Bm*n^2+Bl)-(m*g*d*sin(x2)))/(Jl+Jm*n^2);  %dwl/dt 

dx = [f1; f2; f3];

== matlab function ANTIGOcontrolador/PID 1 DOF Discreto/MATLAB Function2 ==
  data: Sp input; us output; Pv input; Con_ini input; Con_out output
function [us, Con_out] = fcn(Sp, Pv, Con_ini)

en_1 = Con_ini(1);
I_error_1 = Con_ini(2);
difact = Con_ini(3);
Ad_1 = Con_ini(4);
us_1 = Con_ini(5);

umin = -100;
umax = 100;

Kp = 12.194801852041582;
Ki = 1.836264365827931;
Kd = 58.215749090323079;
N = 0.135321750384943;
kaw = 0.1; 

en = Sp - Pv;

if abs(en) > abs(Sp*0.065)
    Ap = Kp*en;
    Ad = Kd*(en-en_1) + N*Ad_1;
    I_error = en + I_error_1 + kaw*difact;
    Ai = Ki*I_error;
    un = Ap + Ai + Ad;
    us = un;

    if un < umin 
        us = umin;
    end
    if un > umax 
        us = umax;
    end

    en_1 = en;
    I_error_1 = I_error;
    difact = us - un;
    Ad_1 = Ad;
    us_1 = us;

else
    us = us_1; % Asignar el último valor de us
end

Con_out = [en_1; I_error_1; difact; Ad_1; us_1];

% 
% function [us, Con_out] = fcn(Sp, Pv, Con_ini)
% 
% en_1 = Con_ini(1);
% I_error_1 = Con_ini(2);
% difact = Con_ini(3);
% Ad_1 = Con_ini(4);
% us_1 = Con_ini(5);
% 
% umin = -100;
% umax = 100;
% 
% Kp = 12.194801852041582;
% Ki = 1.836264365827931;
% Kd = 58.215749090323079;
% N = 0.135321750384943;
% kaw = 0.1; 
% 
% en = Sp - Pv;
% 
%     Ap = Kp*en;
%     Ad = Kd*(en-en_1) + N*Ad_1;
%     I_error = en + I_error_1 + kaw*difact;
%     Ai = Ki*I_error;
%     un = Ap + Ai + Ad;
%     us = un;
% 
%     if un < umin 
%         us = umin;
%     end
%     if un > umax 
%         us = umax;
%     end
% 
%     en_1 = en;
%     I_error_1 = I_error;
%     difact = us - un;
%     Ad_1 = Ad;
%     us_1 = us;
% 
% 
% 
% Con_out = [en_1; I_error_1; difact; Ad_1; us_1];

== matlab function ANTIGOcontrolador/PID 2 DOF/Subsystem/MATLAB Function ==
  data: x input; PWM input; dx output; parametros input
function dx = fcn(x,PWM,parametros)

%ESTADOS
x1 = x(1);
x2 = x(2);
x3 = x(3);

%Parametros
R = parametros(1);
L = parametros(2);
Ki = parametros(3);
Kv = parametros(4);
Jm = parametros(5);
Jl = parametros(6);
Bm = parametros(7);
Bl = parametros(8);
n = parametros(9);
g = parametros(10);
d = parametros(11);
m = parametros(12);

%EXPRESIONES
% Jt = Jm*n^2 +Jl;
% f1 = (1/L)*(((7*PWM)/100) - R*x1 - Kv*x2*n);
% f2 = (1/Jt)*(Ki*x1*n - (Bm*n^2 + Bl)*x2 - m*g*d*sin(x3));
% f3 = x2;

% MODELO 2 ESTADOS I TL WL  SALIDA TL WL
f1 = (((7*PWM)/100)-Kv*x3*n-R*x1)/(L); %di/dt
f2 = x3; %d0l/dt = Wl
f3 = ((Ki*x1*n)-x3*(Bm*n^2+Bl)-(m*g*d*sin(x2)))/(Jl+Jm*n^2);  %dwl/dt 

dx = [f1; f2; f3];

== matlab function ANTIGOcontrolador/PID 2 DOF Discreto/MATLAB Function ==
  data: Sp input; us output; Pv input; Con_ini input; Con_out output
% function [us, Con_out] = fcn(Sp, Pv, Con_ini)
%  
% en_1 = Con_ini(1);
% u1_1 = Con_ini(2);
% Pv_1 = Con_ini(3);
% u2_1 = Con_ini(4);
% difact = Con_ini(5);
% umin = -100;
% umax = 100;
% kaw = 0.01; 
%  
% en = Sp - Pv;
% u1 = 0.153958966653420*en_1 + u1_1 + kaw*difact;
% u2 = 22.177058343736231*Pv - 21.573923642220816*(Pv_1) + 0.732201155629244*u2_1;
% un = u1-u2;
% us = un;
%  
% if un < umin 
%     us = umin;
% end
% if un > umax 
%     us = umax;
% end
%  
% en_1 = en;
% u1_1 = u1;
% Pv_1 = Pv;
% u2_1 = u2;
% difact = us - un;
%          
% Con_out = [en_1; u1_1; Pv_1;u2_1; difact];

function [us, Con_out] = fcn(Sp, Pv, Con_ini)

en_1 = Con_ini(1);
yn_1 = Con_ini(2);
I_error_1 = Con_ini(3);
difact = Con_ini(4);
Ad_1 = Con_ini(5);
Ad1_ = Con_ini(6);

umin = -100;
umax = 100;

Kp = -3.357670445385118;
Ki = 3.822951239710286;
Kd = 32.464560395668343;
N = 0.782109908780621;
Kpd = 0.285776886757601;
Kdp = 3.408050560944484;
N1 = 0.997168715666942;
Ka= 0.1; 

en =  Sp - Pv;
Ap = Kp*en;
Ad = Kd*(en-en_1) + N*Ad1_;
I_error = en + I_error_1 + Ka*difact;
Ai = Ki*I_error;
U1 = Ap + Ai + Ad;

Ap1 = Kpd * Pv;
Ad1 = Kdp * (Pv - yn_1) + N1*Ad_1;
U2 = Ap1 + Ad1;

Uc = U1 - U2;
us = Uc;


if Uc < umin 
    us = umin;
end
if Uc > umax 
    us = umax;
end

en_1 = en;
yn_1 = Pv;
I_error_1 = I_error;
difact = us - Uc;
Ad_1 = Ad1;
Ad1_ = Ad;
      
Con_out = [en_1; yn_1; I_error_1; difact; Ad_1; Ad1_];

== matlab function ANTIGOcontrolador/PID 2 DOF Discreto/Subsystem/MATLAB Function ==
  data: x input; PWM input; dx output; parametros input
function dx = fcn(x,PWM,parametros)

%ESTADOS
x1 = x(1);
x2 = x(2);
x3 = x(3);

%Parametros
R = parametros(1);
L = parametros(2);
Ki = parametros(3);
Kv = parametros(4);
Jm = parametros(5);
Jl = parametros(6);
Bm = parametros(7);
Bl = parametros(8);
n = parametros(9);
g = parametros(10);
d = parametros(11);
m = parametros(12);

%EXPRESIONES
% Jt = Jm*n^2 +Jl;
% f1 = (1/L)*(((7*PWM)/100) - R*x1 - Kv*x2*n);
% f2 = (1/Jt)*(Ki*x1*n - (Bm*n^2 + Bl)*x2 - m*g*d*sin(x3));
% f3 = x2;

% MODELO 2 ESTADOS I TL WL  SALIDA TL WL
f1 = (((7*PWM)/100)-Kv*x3*n-R*x1)/(L); %di/dt
f2 = x3; %d0l/dt = Wl
f3 = ((Ki*x1*n)-x3*(Bm*n^2+Bl)-(m*g*d*sin(x2)))/(Jl+Jm*n^2);  %dwl/dt 

dx = [f1; f2; f3];

== matlab function ANTIGOcontrolador/PID 2 DOF Discreto/MATLAB Function1 ==
  data: Sp input; us output; Pv input; Con_ini input; Con_out output
% function [us, Con_out] = fcn(Sp, Pv, Con_ini)
%  
% en_1 = Con_ini(1);
% u1_1 = Con_ini(2);
% Pv_1 = Con_ini(3);
% u2_1 = Con_ini(4);
% difact = Con_ini(5);
% umin = -100;
% umax = 100;
% kaw = 0.01; 
%  
% en = Sp - Pv;
% u1 = 0.153958966653420*en_1 + u1_1 + kaw*difact;
% u2 = 22.177058343736231*Pv - 21.573923642220816*(Pv_1) + 0.732201155629244*u2_1;
% un = u1-u2;
% us = un;
%  
% if un < umin 
%     us = umin;
% end
% if un > umax 
%     us = umax;
% end
%  
% en_1 = en;
% u1_1 = u1;
% Pv_1 = Pv;
% u2_1 = u2;
% difact = us - un;
%          
% Con_out = [en_1; u1_1; Pv_1;u2_1; difact];

function [us, Con_out] = fcn(Sp, Pv, Con_ini)

en_1 = Con_ini(1);
yn_1 = Con_ini(2);
I_error_1 = Con_ini(3);
difact = Con_ini(4);
Ad_1 = Con_ini(5);
Ad1_ = Con_ini(6);

umin = -100;
umax = 100;

% Kp = 0.01357670445385118;
% Ki = 1.822951239710286;
% Kd = 10.464560395668343;
% N = 0.782109908780621;
% Kpd = 1.285776886757601;
% Kdp = 13.408050560944484;
% N1 = 0.997168715666942;
% Ka= 0.1;

Kp = -3.357670445385118;
Ki = 3.822951239710286;
Kd = 32.464560395668343;
N = 0.782109908780621;
Kpd = 0.285776886757601;
Kdp = 3.408050560944484;
N1 = 0.997168715666942;
Ka= 0.1; 

en =  Sp - Pv;
Ap = Kp*en;
Ad = Kd*(en-en_1) + N*Ad1_;
I_error = en + I_error_1 + Ka*difact;
Ai = Ki*I_error;
U1 = Ap + Ai + Ad;

Ap1 = Kpd * Pv;
Ad1 = Kdp * (Pv - yn_1) + N1*Ad_1;
U2 = Ap1 + Ad1;

Uc = U1 - U2;
us = Uc;


if Uc < umin 
    us = umin;
end
if Uc > umax 
    us = umax;
end

en_1 = en;
yn_1 = Pv;
I_error_1 = I_error;
difact = us - Uc;
Ad_1 = Ad1;
Ad1_ = Ad;
      
Con_out = [en_1; yn_1; I_error_1; difact; Ad_1; Ad1_];

== matlab function ANTIGOcontrolador/Estados Discreto/MATLAB Function1 ==
  data: Sp input; us output; X_est input; Con_ini input; Con_out output
function [us,Con_out] = fcn(Sp,X_est,Con_ini)

umax = 100;
umin = -100;
kaw = zeros(1);
CL = [1, 0]
Ki = [13.038404810405284];
Kes = [8.39272964861829,6.19627625077861];

Vk_1 = Con_ini(1);
dif_act = Con_ini(2);

Tm = 0.03;
Kid = Ki*Tm;

Pv = CL*X_est;
en = Sp - Pv;
Vk = en + Vk_1 + kaw*dif_act;
un = Kid*Vk - Kes*X_est;
us = un;

Vk_1 = Vk;

if un>umax
    us = umax;
end
if un<umin
    us = umin;
end

dif_act = us - un;
Con_out = [Vk_1; dif_act];

== matlab function ANTIGOcontrolador/PID Cascada Discreto/MATLAB Function1 ==
  data: Sp input; u2 output; Pv input; Pv1 input; Con_ini input; Con_out output
function [u2,Con_out] = fcn(Sp,Pv,Pv1,Con_ini)

en_1 = Con_ini(1);
u1_1 = Con_ini(2);
en2_1 = Con_ini(3);
u2_1 = Con_ini(4);

en = Sp - Pv;
u1 = 0.439531738224972*en + 0.093106585918219*en_1+1*u1_1;
en_1 = en;
u1_1 = u1;

u1min = -40;
u1max = 40;

if u1_1 < u1min 
    u1 = u1min;
end
if u1_1 > u1max 
    u1 = u1max;
end

en2 = u1 - Pv1;
u2 = 0*en2 + 93.138459952280698*en2_1+1*u2_1;
en2_1 = en2;
u2_1 = u2;

u2min = -100;
u2max = 100;

if u2_1 < u2min 
    u2 = u2min;
end
if u2_1 > u2max 
    u2 = u2max;
end

Con_out = [en_1; u1_1; en2_1; u2_1];

== matlab function ANTIGOcontrolador/PID Cascada Discreto/MATLAB Function ==
  data: Sp input; u2 output; Pv input; Pv1 input; Con_ini input; Con_out output
function [u2,Con_out] = fcn(Sp,Pv,Pv1,Con_ini)

en_1 = Con_ini(1);
u1_1 = Con_ini(2);
en2_1 = Con_ini(3);
u2_1 = Con_ini(4);

en = Sp - Pv;
u1 = 0.439531738224972*en + 0.093106585918219*en_1+1*u1_1;
en_1 = en;
u1_1 = u1;

u1min = -40;
u1max = 40;

if u1_1 < u1min 
    u1 = u1min;
end
if u1_1 > u1max 
    u1 = u1max;
end

en2 = u1 - Pv1;
u2 = 0*en2 + 93.138459952280698*en2_1+1*u2_1;
en2_1 = en2;
u2_1 = u2;

u2min = -100;
u2max = 100;

if u2_1 < u2min 
    u2 = u2min;
end
if u2_1 > u2max 
    u2 = u2max;
end

Con_out = [en_1; u1_1; en2_1; u2_1];

== matlab function ANTIGOcontrolador/PID Cascada/Subsystem1/MATLAB Function ==
  data: x input; PWM input; dx output; parametros input
function dx = fcn(x,PWM,parametros)

%ESTADOS
x1 = x(1);
x2 = x(2);
x3 = x(3);

%Parametros
R = parametros(1);
L = parametros(2);
Ki = parametros(3);
Kv = parametros(4);
Jm = parametros(5);
Jl = parametros(6);
Bm = parametros(7);
Bl = parametros(8);
n = parametros(9);
g = parametros(10);
d = parametros(11);
m = parametros(12);

%EXPRESIONES
% Jt = Jm*n^2 +Jl;
% f1 = (1/L)*(((7*PWM)/100) - R*x1 - Kv*x2*n);
% f2 = (1/Jt)*(Ki*x1*n - (Bm*n^2 + Bl)*x2 - m*g*d*sin(x3));
% f3 = x2;

% MODELO 2 ESTADOS I TL WL  SALIDA TL WL
f1 = (((7*PWM)/100)-Kv*x3*n-R*x1)/(L); %di/dt
f2 = x3; %d0l/dt = Wl
f3 = ((Ki*x1*n)-x3*(Bm*n^2+Bl)-(m*g*d*sin(x2)))/(Jl+Jm*n^2);  %dwl/dt 

dx = [f1; f2; f3];
